simulink model "p2_vav"  (R2023a)
settings: Solver=VariableStepAuto  StartTime=0.0  StopTime=10.0  RelTol=1e-3
settings Model: Creator=Amirali  LastModifiedBy=Amirali

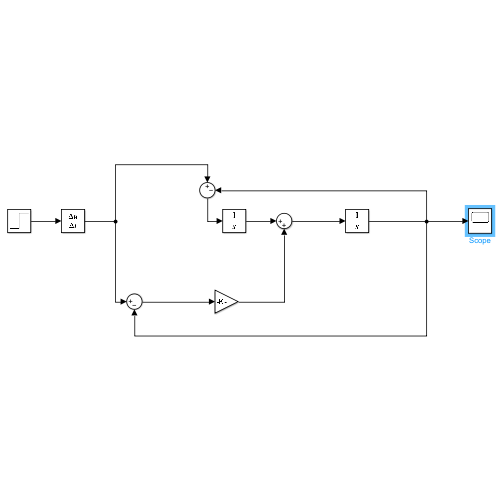
[thumbnail: Simulink's stored preview of the top-level diagram]
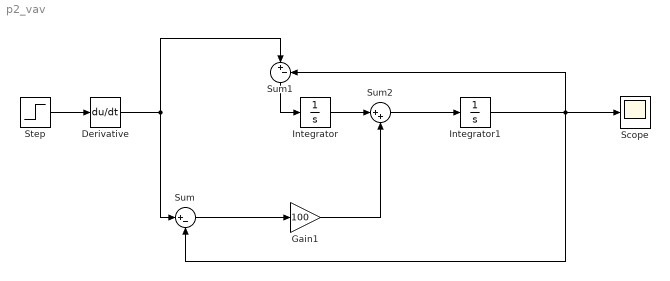
== system p2_vav ==
  Derivative : Derivative
  Gain1 : Gain  Gain=100
  Integrator : Integrator
  Integrator1 : Integrator
  Scope : Scope
  Step : Step  Time=0.001  SampleTime=0
  Sum : Sum  Inputs=|+-
  Sum1 : Sum  Inputs=|+-
  Sum2 : Sum  Inputs=|++
  wires:
  Sum/1 -> Gain1/1
  Step/1 -> Derivative/1
  Integrator/1 -> Sum2/1
  Integrator1/1 -> Scope/1, Sum1/2, Sum/2
  Derivative/1 -> Sum1/1, Sum/1
  Sum2/1 -> Integrator1/1
  Sum1/1 -> Integrator/1
  Gain1/1 -> Sum2/2
